simulink model "combinational_logic"  (R2019a)
settings: Solver=VariableStepAuto  StartTime=0.0  StopTime=2  MaxStep=0.02  RelTol=1e-3
settings Model: Creator=何泽楷  LastModifiedBy=何泽楷
settings OptimizationCC: BooleanDataType=off

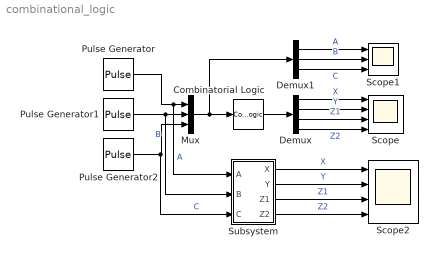
== system combinational_logic ==
  Combinatorial Logic : CombinatorialLogic  TruthTable=[1, 1, 1, 1; 1, 0, 1, 0; 1, 0, 1, 0; 1, 0, 1, 0; 1, 0, 1, 0; 1, 0, 1, 0; 1, 0, 1, 0; 0, 1, 1, 0];
  Demux : Demux
  Demux1 : Demux  Outputs=3
  Mux : Mux  Inputs=3
  Pulse Generator : DiscretePulseGenerator  PhaseDelay=1  SampleTime=0.1
  Pulse Generator1 : DiscretePulseGenerator  Period=4  PulseWidth=2  PhaseDelay=2  SampleTime=0.1
  Pulse Generator2 : DiscretePulseGenerator  Period=8  PulseWidth=4  PhaseDelay=4  SampleTime=0.1
  Scope : Scope  NumInputPorts=4
  Scope1 : Scope  NumInputPorts=3
  Scope2 : Scope  NumInputPorts=4
  Subsystem : Subsystem
      mask help: Subsystem for Problem 1, Chapter 6. The input X, Y, Z are logical varibales, output X= ~(AB) + ~(BC) + ~(CA), Y = (~A + B)(~B + C)(~C + A); Z1 = X + Y, Z2 = XY.
  wires:
  Pulse Generator/1 -> Subsystem/1(A), Mux/1  "A"
  Mux/1 -> Demux1/1, Combinatorial Logic/1
  Pulse Generator1/1 -> Subsystem/2(B), Mux/2  "B"
  Pulse Generator2/1 -> Subsystem/3(C), Mux/3  "C"
  Combinatorial Logic/1 -> Demux/1
  Demux/2 -> Scope/2  "Y"
  Demux/3 -> Scope/3  "Z1"
  Demux/4 -> Scope/4  "Z2"
  Demux1/1 -> Scope1/1  "A"
  Demux1/2 -> Scope1/2  "B"
  Demux1/3 -> Scope1/3  "C"
  Demux/1 -> Scope/1  "X"
  Subsystem/1(X) -> Scope2/1  "X"
  Subsystem/2(Y) -> Scope2/2  "Y"
  Subsystem/3(Z1) -> Scope2/3  "Z1"
  Subsystem/4(Z2) -> Scope2/4  "Z2"

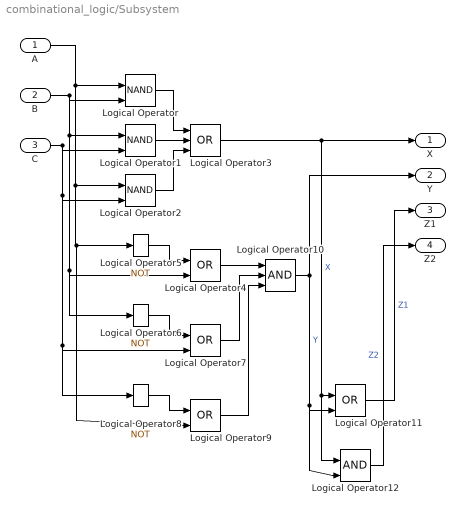
== system combinational_logic/Subsystem ==
  A : Inport
  B : Inport  Port=2
  C : Inport  Port=3
  Logical Operator : Logic  Operator=NAND  IconShape=distinctive  AllPortsSameDT=off  OutDataTypeStr=boolean
  Logical Operator1 : Logic  Operator=NAND  IconShape=distinctive  AllPortsSameDT=off  OutDataTypeStr=boolean
  Logical Operator10 : Logic  Inputs=3  IconShape=distinctive  AllPortsSameDT=off  OutDataTypeStr=boolean
  Logical Operator{4,7,9,11} (4 alike) : Logic  Operator=OR  IconShape=distinctive  AllPortsSameDT=off  OutDataTypeStr=boolean
  Logical Operator12 : Logic  IconShape=distinctive  AllPortsSameDT=off  OutDataTypeStr=boolean
  Logical Operator2 : Logic  Operator=NAND  IconShape=distinctive  AllPortsSameDT=off  OutDataTypeStr=boolean
  Logical Operator3 : Logic  Operator=OR  Inputs=3  IconShape=distinctive  AllPortsSameDT=off  OutDataTypeStr=boolean
  Logical Operator5 : Logic  Operator=NOT  IconShape=distinctive  AllPortsSameDT=off  OutDataTypeStr=boolean
  Logical Operator6 : Logic  Operator=NOT  IconShape=distinctive  AllPortsSameDT=off  OutDataTypeStr=boolean
  Logical Operator8 : Logic  Operator=NOT  IconShape=distinctive  AllPortsSameDT=off  OutDataTypeStr=boolean
  X : Outport
  Y : Outport  Port=2
  Z1 : Outport  Port=3
  Z2 : Outport  Port=4
  wires:
  C/1 -> Logical Operator8/1, Logical Operator7/2, Logical Operator2/2, Logical Operator1/2
  Logical Operator/1 -> Logical Operator3/1
  Logical Operator10/1 -> Y/1, Logical Operator12/2, Logical Operator11/2  "Y"
  Logical Operator2/1 -> Logical Operator3/3
  B/1 -> Logical Operator6/1, Logical Operator4/2, Logical Operator1/1, Logical Operator/2
  Logical Operator3/1 -> X/1, Logical Operator12/1, Logical Operator11/1  "X"
  A/1 -> Logical Operator9/2, Logical Operator5/1, Logical Operator2/1, Logical Operator/1
  Logical Operator7/1 -> Logical Operator10/2
  Logical Operator4/1 -> Logical Operator10/1
  Logical Operator8/1 -> Logical Operator9/1
  Logical Operator12/1 -> Z2/1  "Z2"
  Logical Operator6/1 -> Logical Operator7/1
  Logical Operator5/1 -> Logical Operator4/1
  Logical Operator1/1 -> Logical Operator3/2
  Logical Operator9/1 -> Logical Operator10/3
  Logical Operator11/1 -> Z1/1  "Z1"
